simulink library "intraDynamicSpoolingController_ul"  (R2018b)
settings: Solver=VariableStepAuto  StartTime=0.0  StopTime=10.0  RelTol=1e-3
undefined symbols (not defined in the file or in its folder): pathCtrl
libraries: firstOrderFilter_ul x1
settings Model: Creator=James Reed  LastModifiedBy=jldanie5

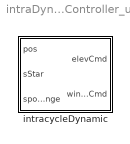
== system intraDynamicSpoolingController_ul ==
  intracycleDynamic : Subsystem

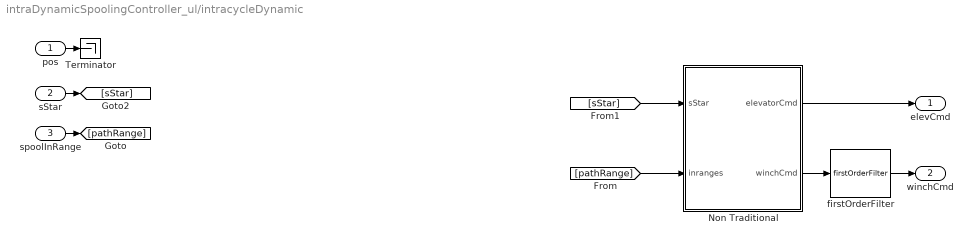
== system intraDynamicSpoolingController_ul/intracycleDynamic ==
  pos : Inport
  "sStar " : Inport  Port=2
  spoolInRange : Inport  Port=3
  Non Traditional : Stateflow chart  TreatAsAtomicUnit=on  mask{reelInSpd=pathCtrl.winchSpeedIn.Value, reelOutSpd=pathCtrl.winchSpeedOut.Value, elevatorReelInDef=pathCtrl.elevatorReelInDef.Value}
      mask prompts: reelInSpd "Reel in speed"; reelOutSpd "Reel out speed"; elevatorReelInDef "Elevator deflection during reel in"
  Terminator : Terminator
  firstOrderFilter : firstOrderFilter_ul/firstOrderFilter  tau=1  ic=0
  elevCmd : Outport
  "winchCmd " : Outport  Port=2
  wires:
  firstOrderFilter/1 -> "winchCmd "/1
  Non Traditional/1(elevatorCmd) -> elevCmd/1
  Non Traditional/2(winchCmd) -> firstOrderFilter/1
  pos/1 -> Terminator/1
  [sStar] -> Non Traditional/1(sStar)
  "sStar "/1 -> [sStar]
  spoolInRange/1 -> [pathRange]
  [pathRange] -> Non Traditional/2(inranges)

== stateflow chart intraDynamicSpoolingController_ul/intracycleDynamic/Non Traditional ==
  state ReelIn
    entry:
    elevatorCmd= elevatorReelInDef;
    winchCmd = reelInSpd;
  state ReelOut
    entry:
    winchCmd = reelOutSpd;
    elevatorCmd= 0;
  (default) -> ReelOut
  ReelIn -> ReelOut : [ ~any(and(sStar>=inranges(:,1),sStar<inranges(:,2)))]
  ReelOut -> ReelIn : [any(and(sStar>=inranges(:,1),sStar<inranges(:,2)))]
  data: elevatorCmd output; sStar input; winchCmd output; inranges input; reelInSpd parameter; reelOutSpd parameter; elevatorReelInDef parameter
